simulink model "modello_carroponte_controllo"  (R2023b)
settings: Solver=FixedStepAuto  StartTime=0  StopTime=30  FixedStep=1e-3  RelTol=1e-3  EnableMultiTasking=on
values from neighbouring files (symbols this model uses):
  alpha_0 = 80 * pi/180    (= 1.3962634016)    [carroponte_controllo.m]
  alpha_dot_0 = 0    [carroponte_controllo.m]
  C = 5000 * Numerator/Denominator    [carroponte_controllo.m]
  cc = 5000    [carroponte_controllo.m]
  cm = 100    [carroponte_controllo.m]
  g = 9.81    [carroponte_controllo.m]
  L = 2.5    [carroponte_controllo.m]
  mc = 300    [carroponte_controllo.m]
  mm = 1000    [carroponte_controllo.m]
  xc_0 = 0    [carroponte_controllo.m]
  xc_dot_0 = 0    [carroponte_controllo.m]
libraries: slpidlib x1
settings Model: Creator=Gianmarco Rallo  LastModifiedBy=andrearosini
settings SolverCC: AlgebraicLoopSolver=TrustRegion
settings DataIOCC: LimitDataPoints=on  ReturnWorkspaceOutputs=off
settings OptimizationCC: BlockReduction=off  DefaultParameterBehavior=Inlined  BufferReuse=off  LifeSpan=inf
settings DebuggingCC: UnconnectedInputMsg=warning  UnconnectedOutputMsg=warning  UnconnectedLineMsg=warning  AllowSymbolicDim=off  SFUnexpectedBacktrackingDiag=warning  SFNoUnconditionalDefaultTransitionDiag=warning  SFExecutionAtInitializationDiag=none  ArithmeticOperatorsInVariantConditions=warning
settings ModelReferenceCC: EnableRefExpFcnMdlSchedulingChecks=on  PropagateSignalLabelsOutOfModel=off
settings SFSimCC: SimUseLocalCustomCode=off  CustomCodeUndefinedFunction=UseInterfaceOnly
settings RTWCC: RTWUseLocalCustomCode=off
settings CodeAppCC: StateflowObjectComments=on
settings GRTTargetCC: TargetLangStandard=C89/C90 (ANSI)
settings ConfigComp: CovMetricSettings=dw  CovSaveCumulativeToWorkspaceVar=on  CovSaveSingleToWorkspaceVar=on  CovExternalEMLEnable=off

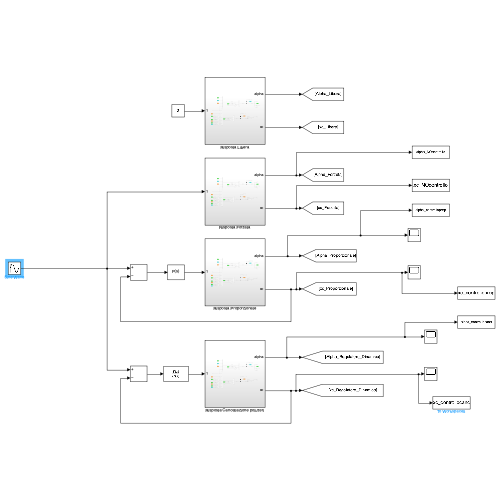
[thumbnail: Simulink's stored preview of the top-level diagram]
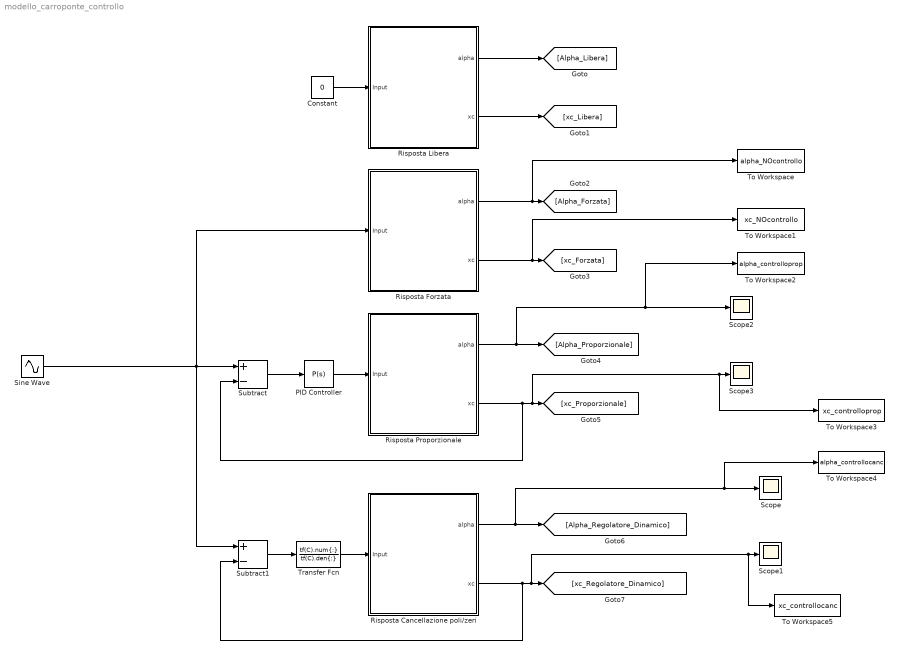
== system modello_carroponte_controllo ==
  Constant : Constant  Value=0
  PID Controller : slpidlib/PID Controller  Controller=P  Form=Parallel  TimeDomain=Continuous-time  UseExternalTs=off  SampleTime=-1  IntegratorMethod=Forward Euler  FilterMethod=Forward Euler  ControllerParametersSource=internal  P=5e3  I=1  UseKiTs=off  D=0  N=100  UseFilter=on  TunerSelectOption=Transfer Function Based (PID Tuner App)  InitialConditionSource=internal  InitialConditionForIntegrator=0  InitialConditionForFilter=0  DifferentiatorICPrevScaledInput=0  ExternalReset=none  TrackingMode=off  Kt=1  LimitOutput=off  SatLimitsSource=internal  UpperSaturationLimit=inf  LowerSaturationLimit=-inf  LinearizeAsGain=on  AntiWindupMode=none  Kb=1  LimitIntegrator=off  UpperIntegratorSaturationLimit=inf  LowerIntegratorSaturationLimit=-inf  POutMin=[]  POutMax=[]  IOutMin=[]  IOutMax=[]  DOutMin=[]  DOutMax=[]  NOutMin=[]  NOutMax=[]  SumOutMin=[]  SumOutMax=[]  SaturationOutMin=[]  SaturationOutMax=[]  PParamMin=[]  PParamMax=[]  IParamMin=[]  IParamMax=[]  DParamMin=[]  DParamMax=[]  NParamMin=[]  NParamMax=[]  KbParamMin=[]  KbParamMax=[]  KtParamMin=[]  KtParamMax=[]  KbOutMin=[]  KbOutMax=[]  KtOutMin=[]  KtOutMax=[]  IntegratorOutMin=[]  IntegratorOutMax=[]  FilterOutMin=[]  FilterOutMax=[]  SumI1OutMin=[]  SumI1OutMax=[]  SumI2OutMin=[]  SumI2OutMax=[]  SumI3OutMin=[]  SumI3OutMax=[]  SumI4OutMin=[]  SumI4OutMax=[]  SumDOutMin=[]  SumDOutMax=[]  DifferentiatorOutMin=[]  DifferentiatorOutMax=[]  FilterDiffOutCoefMin=[]  FilterDiffOutCoefMax=[]  ReciprocalOutMin=[]  ReciprocalOutMax=[]  SumDenOutMin=[]  SumDenOutMax=[]  SumNumOutMin=[]  SumNumOutMax=[]  DivideOutMin=[]  DivideOutMax=[]  UdiffTsProdOutMin=[]  UdiffTsProdOutMax=[]  NTsProdOutMin=[]  NTsProdOutMax=[]  UintegralTsProdOutMin=[]  UintegralTsProdOutMax=[]  UngainTsProdOutMin=[]  UngainTsProdOutMax=[]  ClampingZeroOutDataTypeStr=Inherit: Inherit via back propagation  ClampingZeroOutMin=[]  ClampingZeroOutMax=[]  FilterDenConstantOutDataTypeStr=Inherit: Inherit via back propagation  FilterDenConstantOutMin=[]  FilterDenConstantOutMax=[]  PCopyOutDataTypeStr=Inherit: Inherit via back propagation  PCopyOutMin=[]  PCopyOutMax=[]  NCopyOutDataTypeStr=Inherit: Inherit via back propagation  NCopyOutMin=[]  NCopyOutMax=[]  IntegratorContinuousStateAttributes=''  IntegratorStateMustResolveToSignalObject=off  IntegratorRTWStateStorageClass=Auto  FilterContinuousStateAttributes=''  FilterStateMustResolveToSignalObject=off  FilterRTWStateStorageClass=Auto  ParallelPVariant=InternalParameters  IdealPVariant=Disabled  IVariant=Disabled  DVariant=Disabled  IntegratorVariant=Disabled  SatVariant=Disabled  AWVariant=Disabled  PCopyVariant=Disabled  TRVariant=Disabled  FdbkBlocksVariant=Forward  IdealPFdbkVariant=Disabled  SatFdbkVariant=Disabled  DerivativeFilterVariant=Disabled  NVariant=Disabled  NCopyVariant=Disabled_SignalSpec  FilterICVariant=Disabled  IntegratorICVariant=Disabled  ExternalResetVariant=Disabled  TRSumVariant=Passthrough  SumFdbkVariant=Disabled  SumVariant=Passthrough_P  TsampFilterVariant=InternalTs  TsampNgainVariant=Passthrough  TsampIntegralVariant=Disabled_SignalSpec  ExternalSaturationOutDataTypeStr=Inherit: Same as second input
  Risposta Cancellazione poli/zeri : Subsystem
  Risposta Forzata : Subsystem
  Risposta Libera : Subsystem
  Risposta Proporzionale : Subsystem
  Scope{,1..3} (4 alike) : Scope
  Sine Wave : Sin  Amplitude=0  Frequency=2  SampleTime=0
  Subtract : Sum  Inputs=+-
  Subtract1 : Sum  Inputs=+-
  To Workspace : ToWorkspace  VariableName=alpha_NOcontrollo  SaveFormat=Timeseries  SampleTime=-1
  To Workspace1 : ToWorkspace  VariableName=xc_NOcontrollo  SaveFormat=Timeseries  SampleTime=-1
  To Workspace2 : ToWorkspace  VariableName=alpha_controlloprop  SaveFormat=Timeseries  SampleTime=-1
  To Workspace3 : ToWorkspace  VariableName=xc_controlloprop  SaveFormat=Timeseries  SampleTime=-1
  To Workspace4 : ToWorkspace  VariableName=alpha_controllocanc  SaveFormat=Timeseries  SampleTime=-1
  To Workspace5 : ToWorkspace  VariableName=xc_controllocanc  SaveFormat=Timeseries  SampleTime=-1
  Transfer Fcn : TransferFcn  Numerator=tf(C).num{:}  Denominator=tf(C).den{:}
  wires:
  Risposta Libera/1(alpha) -> [Alpha_Libera]
  Risposta Libera/2(xc) -> [xc_Libera]
  Constant/1 -> Risposta Libera/1(Input)
  Risposta Forzata/2(xc) -> To Workspace1/1, [xc_Forzata]
  Risposta Forzata/1(alpha) -> To Workspace/1, [Alpha_Forzata]
  Risposta Proporzionale/1(alpha) -> To Workspace2/1, Scope2/1, [Alpha_Proporzionale]
  Risposta Proporzionale/2(xc) -> Subtract/2, To Workspace3/1, Scope3/1, [xc_Proporzionale]
  PID Controller/1 -> Risposta Proporzionale/1(Input)
  Subtract/1 -> PID Controller/1
  Sine Wave/1 -> Risposta Forzata/1(Input), Subtract1/1, Subtract/1
  Subtract1/1 -> Transfer Fcn/1
  Transfer Fcn/1 -> Risposta Cancellazione poli/zeri/1(Input)
  Risposta Cancellazione poli/zeri/2(xc) -> To Workspace5/1, Scope1/1, [xc_Regolatore_Dinamico], Subtract1/2
  Risposta Cancellazione poli/zeri/1(alpha) -> To Workspace4/1, Scope/1, [Alpha_Regolatore_Dinamico]

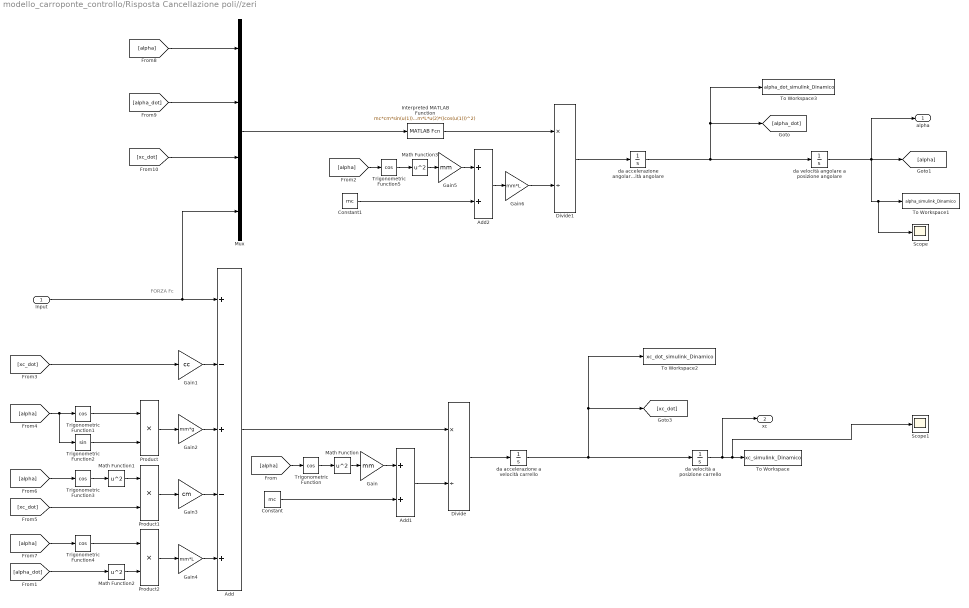
== system modello_carroponte_controllo/Risposta Cancellazione poli//zeri ==
  note: FORZA Fc
  Input : Inport
  Add : Sum  Inputs=+-+-+
  Add1 : Sum
  Add2 : Sum
  Constant : Constant  Value=mc
  Constant1 : Constant  Value=mc
  Divide : Product  Inputs=*/
  Divide1 : Product  Inputs=*/
  Gain : Gain  Gain=mm
  Gain1 : Gain  Gain=cc
  Gain2 : Gain  Gain=mm*g
  Gain3 : Gain  Gain=cm
  Gain4 : Gain  Gain=mm*L
  Gain5 : Gain  Gain=mm
  Gain6 : Gain  Gain=mm*L
  Interpreted MATLAB Function : MATLABFcn  MATLABFcn=mc*cm*sin(u(1))*u(3) - mm*cc*sin(u(1))*u(3) + (mm^2)*L*sin(u(1))*cos(u(1))*(u(2)^2) + mm*sin(u(1))*u(4) + (mm^2)*g*cos(u(1)) + mc*mm*g*cos(u(1)) - mc*cm*L*u(2) - mm*cm*L*u(2)*((cos(u(1)))^2)  OutputDimensions=1
  Math Function{,1..3} (4 alike) : Math  Operator=square  SignedPower=on
  Mux : Mux
  Product : Product
  Product1 : Product
  Product2 : Product
  Scope : Scope
  Scope1 : Scope
  To Workspace : ToWorkspace  VariableName=xc_simulink_Dinamico  SampleTime=-1
  To Workspace1 : ToWorkspace  VariableName=alpha_simulink_Dinamico  SampleTime=-1
  To Workspace2 : ToWorkspace  VariableName=xc_dot_simulink_Dinamico  SampleTime=-1
  To Workspace3 : ToWorkspace  VariableName=alpha_dot_simulink_Dinamico  SampleTime=-1
  Trigonometric Function{,1,3..5} (5 alike) : Trigonometry  Operator=cos
  Trigonometric Function2 : Trigonometry
  da accelerazione a velocità carrello : Integrator  InitialCondition=xc_dot_0
  da accelerazione angolare a velocità angolare : Integrator  InitialCondition=alpha_dot_0
  da velocità a posizione carrello : Integrator  InitialCondition=xc_0
  da velocità angolare a posizione angolare : Integrator  InitialCondition=alpha_0
  alpha : Outport
  xc : Outport  Port=2
  wires:
  Math Function2/1 -> Product2/2
  [alpha] -> Trigonometric Function4/1
  Gain4/1 -> Add/5
  [xc_dot] -> Mux/3
  Trigonometric Function3/1 -> Math Function1/1
  [alpha_dot] -> Math Function2/1
  Gain3/1 -> Add/4
  Product1/1 -> Gain3/1
  Gain6/1 -> Divide1/2
  Gain2/1 -> Add/3
  Divide/1 -> da accelerazione a velocità carrello/1
  [alpha_dot] -> Mux/2
  Input/1 -> Add/1, Mux/4
  [xc_dot] -> Gain1/1
  da velocità a posizione carrello/1 -> To Workspace/1, Scope1/1, xc/1
  Product2/1 -> Gain4/1
  Trigonometric Function/1 -> Math Function/1
  Product/1 -> Gain2/1
  Add2/1 -> Gain6/1
  Divide1/1 -> da accelerazione angolare a velocità angolare/1
  Interpreted MATLAB Function/1 -> Divide1/1
  Trigonometric Function4/1 -> Product2/1
  Gain5/1 -> Add2/1
  Trigonometric Function1/1 -> Product/1
  [alpha] -> Trigonometric Function5/1
  Gain1/1 -> Add/2
  Trigonometric Function5/1 -> Math Function3/1
  Add1/1 -> Divide/2
  Constant1/1 -> Add2/2
  Add/1 -> Divide/1
  Math Function3/1 -> Gain5/1
  Mux/1 -> Interpreted MATLAB Function/1
  Constant/1 -> Add1/2
  [alpha] -> Trigonometric Function1/1, Trigonometric Function2/1
  [xc_dot] -> Product1/2
  Math Function1/1 -> Product1/1
  Trigonometric Function2/1 -> Product/2
  da accelerazione angolare a velocità angolare/1 -> da velocità angolare a posizione angolare/1, [alpha_dot], To Workspace3/1
  [alpha] -> Trigonometric Function/1
  da accelerazione a velocità carrello/1 -> [xc_dot], To Workspace2/1, da velocità a posizione carrello/1
  [alpha] -> Mux/1
  [alpha] -> Trigonometric Function3/1
  Math Function/1 -> Gain/1
  Gain/1 -> Add1/1
  da velocità angolare a posizione angolare/1 -> [alpha], To Workspace1/1, Scope/1, alpha/1

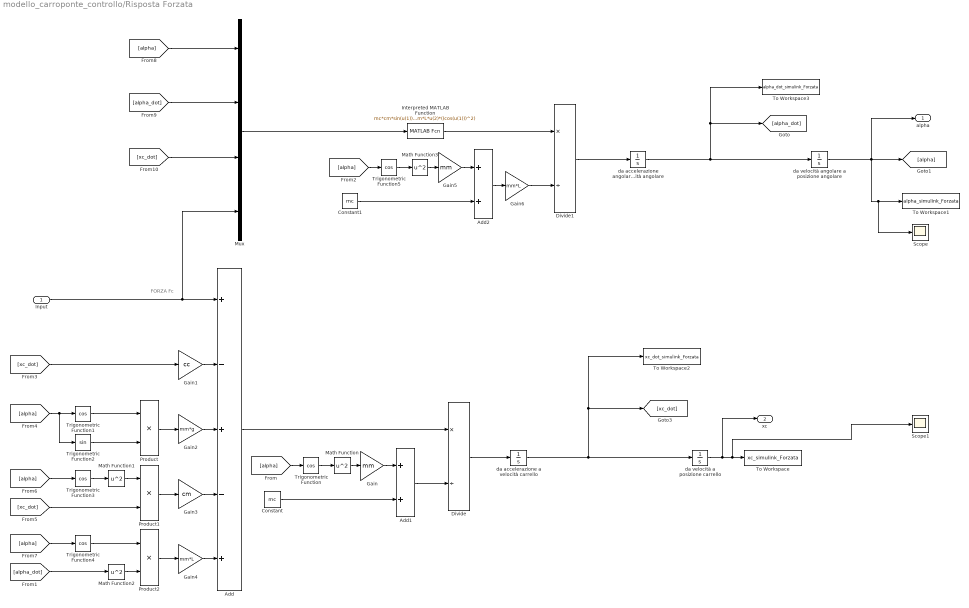
== system modello_carroponte_controllo/Risposta Forzata ==
  note: FORZA Fc
  Input : Inport
  Add : Sum  Inputs=+-+-+
  Add1 : Sum
  Add2 : Sum
  Constant : Constant  Value=mc
  Constant1 : Constant  Value=mc
  Divide : Product  Inputs=*/
  Divide1 : Product  Inputs=*/
  Gain : Gain  Gain=mm
  Gain1 : Gain  Gain=cc
  Gain2 : Gain  Gain=mm*g
  Gain3 : Gain  Gain=cm
  Gain4 : Gain  Gain=mm*L
  Gain5 : Gain  Gain=mm
  Gain6 : Gain  Gain=mm*L
  Interpreted MATLAB Function : MATLABFcn  MATLABFcn=mc*cm*sin(u(1))*u(3) - mm*cc*sin(u(1))*u(3) + (mm^2)*L*sin(u(1))*cos(u(1))*(u(2)^2) + mm*sin(u(1))*u(4) + (mm^2)*g*cos(u(1)) + mc*mm*g*cos(u(1)) - mc*cm*L*u(2) - mm*cm*L*u(2)*((cos(u(1)))^2)  OutputDimensions=1
  Math Function{,1..3} (4 alike) : Math  Operator=square  SignedPower=on
  Mux : Mux
  Product : Product
  Product1 : Product
  Product2 : Product
  Scope : Scope
  Scope1 : Scope
  To Workspace : ToWorkspace  VariableName=xc_simulink_Forzata  SampleTime=-1
  To Workspace1 : ToWorkspace  VariableName=alpha_simulink_Forzata  SampleTime=-1
  To Workspace2 : ToWorkspace  VariableName=xc_dot_simulink_Forzata  SampleTime=-1
  To Workspace3 : ToWorkspace  VariableName=alpha_dot_simulink_Forzata  SampleTime=-1
  Trigonometric Function{,1,3..5} (5 alike) : Trigonometry  Operator=cos
  Trigonometric Function2 : Trigonometry
  da accelerazione a velocità carrello : Integrator  InitialCondition=xc_dot_0
  da accelerazione angolare a velocità angolare : Integrator  InitialCondition=alpha_dot_0
  da velocità a posizione carrello : Integrator  InitialCondition=xc_0
  da velocità angolare a posizione angolare : Integrator  InitialCondition=alpha_0
  alpha : Outport
  xc : Outport  Port=2
  wires:
  Math Function2/1 -> Product2/2
  [alpha] -> Trigonometric Function4/1
  Gain4/1 -> Add/5
  [xc_dot] -> Mux/3
  Trigonometric Function3/1 -> Math Function1/1
  [alpha_dot] -> Math Function2/1
  Gain3/1 -> Add/4
  Product1/1 -> Gain3/1
  Gain6/1 -> Divide1/2
  Gain2/1 -> Add/3
  Divide/1 -> da accelerazione a velocità carrello/1
  [alpha_dot] -> Mux/2
  Input/1 -> Add/1, Mux/4
  [xc_dot] -> Gain1/1
  da velocità a posizione carrello/1 -> To Workspace/1, Scope1/1, xc/1
  Product2/1 -> Gain4/1
  Trigonometric Function/1 -> Math Function/1
  Product/1 -> Gain2/1
  Add2/1 -> Gain6/1
  Divide1/1 -> da accelerazione angolare a velocità angolare/1
  Interpreted MATLAB Function/1 -> Divide1/1
  Trigonometric Function4/1 -> Product2/1
  Gain5/1 -> Add2/1
  Trigonometric Function1/1 -> Product/1
  [alpha] -> Trigonometric Function5/1
  Gain1/1 -> Add/2
  Trigonometric Function5/1 -> Math Function3/1
  Add1/1 -> Divide/2
  Constant1/1 -> Add2/2
  Add/1 -> Divide/1
  Math Function3/1 -> Gain5/1
  Mux/1 -> Interpreted MATLAB Function/1
  Constant/1 -> Add1/2
  [alpha] -> Trigonometric Function1/1, Trigonometric Function2/1
  [xc_dot] -> Product1/2
  Math Function1/1 -> Product1/1
  Trigonometric Function2/1 -> Product/2
  da accelerazione angolare a velocità angolare/1 -> da velocità angolare a posizione angolare/1, [alpha_dot], To Workspace3/1
  [alpha] -> Trigonometric Function/1
  da accelerazione a velocità carrello/1 -> [xc_dot], To Workspace2/1, da velocità a posizione carrello/1
  [alpha] -> Mux/1
  [alpha] -> Trigonometric Function3/1
  Math Function/1 -> Gain/1
  Gain/1 -> Add1/1
  da velocità angolare a posizione angolare/1 -> [alpha], To Workspace1/1, Scope/1, alpha/1

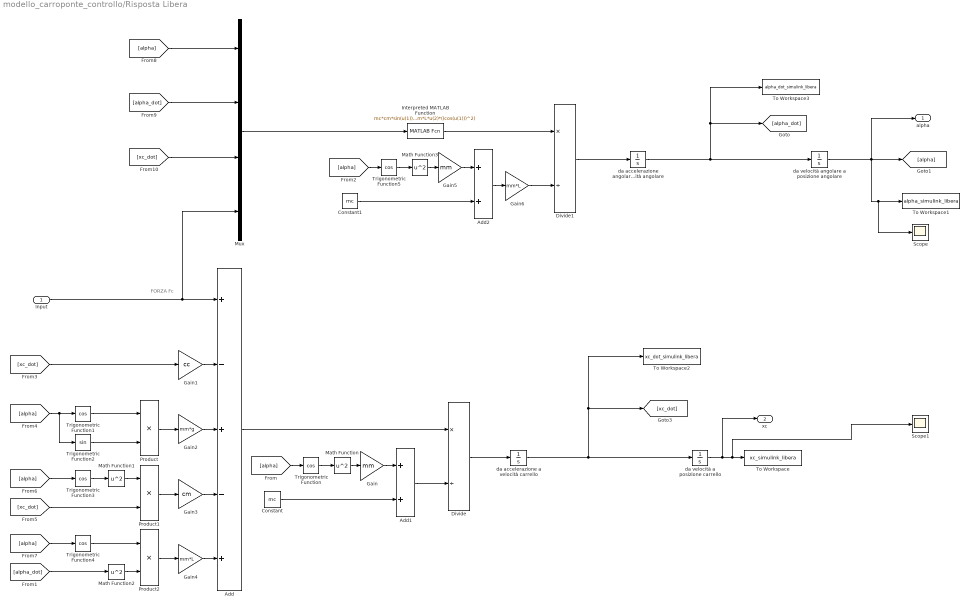
== system modello_carroponte_controllo/Risposta Libera ==
  note: FORZA Fc
  Input : Inport
  Add : Sum  Inputs=+-+-+
  Add1 : Sum
  Add2 : Sum
  Constant : Constant  Value=mc
  Constant1 : Constant  Value=mc
  Divide : Product  Inputs=*/
  Divide1 : Product  Inputs=*/
  Gain : Gain  Gain=mm
  Gain1 : Gain  Gain=cc
  Gain2 : Gain  Gain=mm*g
  Gain3 : Gain  Gain=cm
  Gain4 : Gain  Gain=mm*L
  Gain5 : Gain  Gain=mm
  Gain6 : Gain  Gain=mm*L
  Interpreted MATLAB Function : MATLABFcn  MATLABFcn=mc*cm*sin(u(1))*u(3) - mm*cc*sin(u(1))*u(3) + (mm^2)*L*sin(u(1))*cos(u(1))*(u(2)^2) + mm*sin(u(1))*u(4) + (mm^2)*g*cos(u(1)) + mc*mm*g*cos(u(1)) - mc*cm*L*u(2) - mm*cm*L*u(2)*((cos(u(1)))^2)  OutputDimensions=1
  Math Function{,1..3} (4 alike) : Math  Operator=square  SignedPower=on
  Mux : Mux
  Product : Product
  Product1 : Product
  Product2 : Product
  Scope : Scope
  Scope1 : Scope
  To Workspace : ToWorkspace  VariableName=xc_simulink_libera  SampleTime=-1
  To Workspace1 : ToWorkspace  VariableName=alpha_simulink_libera  SampleTime=-1
  To Workspace2 : ToWorkspace  VariableName=xc_dot_simulink_libera  SampleTime=-1
  To Workspace3 : ToWorkspace  VariableName=alpha_dot_simulink_libera  SampleTime=-1
  Trigonometric Function{,1,3..5} (5 alike) : Trigonometry  Operator=cos
  Trigonometric Function2 : Trigonometry
  da accelerazione a velocità carrello : Integrator  InitialCondition=xc_dot_0
  da accelerazione angolare a velocità angolare : Integrator  InitialCondition=alpha_dot_0
  da velocità a posizione carrello : Integrator  InitialCondition=xc_0
  da velocità angolare a posizione angolare : Integrator  InitialCondition=alpha_0
  alpha : Outport
  xc : Outport  Port=2
  wires:
  da velocità angolare a posizione angolare/1 -> alpha/1, Scope/1, To Workspace1/1, [alpha]
  Gain/1 -> Add1/1
  Math Function/1 -> Gain/1
  [alpha] -> Trigonometric Function3/1
  [alpha] -> Mux/1
  da accelerazione a velocità carrello/1 -> da velocità a posizione carrello/1, To Workspace2/1, [xc_dot]
  [alpha] -> Trigonometric Function/1
  da accelerazione angolare a velocità angolare/1 -> To Workspace3/1, [alpha_dot], da velocità angolare a posizione angolare/1
  Trigonometric Function2/1 -> Product/2
  Math Function1/1 -> Product1/1
  [xc_dot] -> Product1/2
  [alpha] -> Trigonometric Function2/1, Trigonometric Function1/1
  Constant/1 -> Add1/2
  Mux/1 -> Interpreted MATLAB Function/1
  Math Function3/1 -> Gain5/1
  Add/1 -> Divide/1
  Constant1/1 -> Add2/2
  Add1/1 -> Divide/2
  Trigonometric Function5/1 -> Math Function3/1
  Gain1/1 -> Add/2
  [alpha] -> Trigonometric Function5/1
  Trigonometric Function1/1 -> Product/1
  Gain5/1 -> Add2/1
  Trigonometric Function4/1 -> Product2/1
  Interpreted MATLAB Function/1 -> Divide1/1
  Divide1/1 -> da accelerazione angolare a velocità angolare/1
  Add2/1 -> Gain6/1
  Product/1 -> Gain2/1
  Trigonometric Function/1 -> Math Function/1
  Product2/1 -> Gain4/1
  da velocità a posizione carrello/1 -> xc/1, Scope1/1, To Workspace/1
  [xc_dot] -> Gain1/1
  Input/1 -> Mux/4, Add/1
  [alpha_dot] -> Mux/2
  Divide/1 -> da accelerazione a velocità carrello/1
  Gain2/1 -> Add/3
  Gain6/1 -> Divide1/2
  Product1/1 -> Gain3/1
  Gain3/1 -> Add/4
  [alpha_dot] -> Math Function2/1
  Trigonometric Function3/1 -> Math Function1/1
  [xc_dot] -> Mux/3
  Gain4/1 -> Add/5
  [alpha] -> Trigonometric Function4/1
  Math Function2/1 -> Product2/2

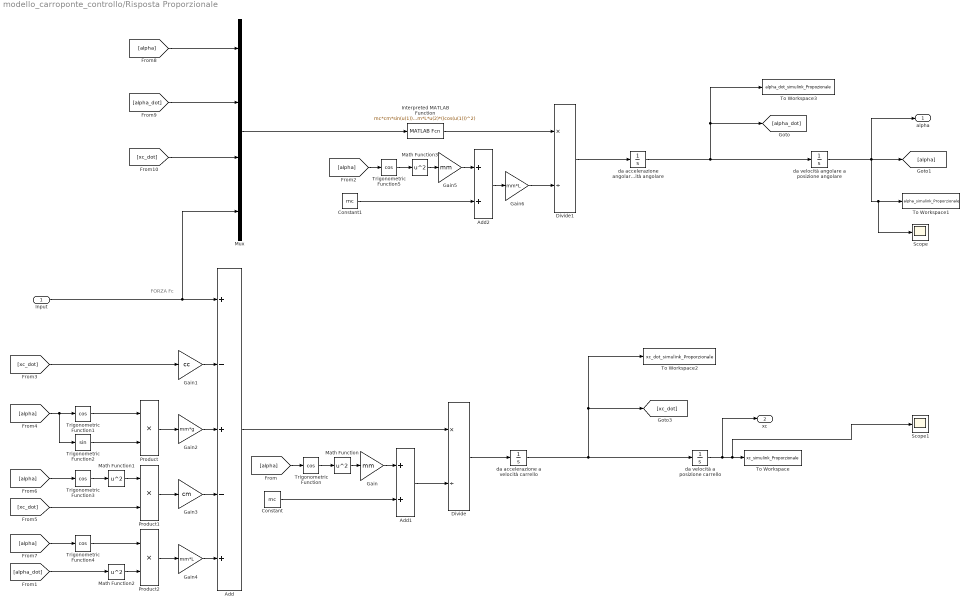
== system modello_carroponte_controllo/Risposta Proporzionale ==
  note: FORZA Fc
  Input : Inport
  Add : Sum  Inputs=+-+-+
  Add1 : Sum
  Add2 : Sum
  Constant : Constant  Value=mc
  Constant1 : Constant  Value=mc
  Divide : Product  Inputs=*/
  Divide1 : Product  Inputs=*/
  Gain : Gain  Gain=mm
  Gain1 : Gain  Gain=cc
  Gain2 : Gain  Gain=mm*g
  Gain3 : Gain  Gain=cm
  Gain4 : Gain  Gain=mm*L
  Gain5 : Gain  Gain=mm
  Gain6 : Gain  Gain=mm*L
  Interpreted MATLAB Function : MATLABFcn  MATLABFcn=mc*cm*sin(u(1))*u(3) - mm*cc*sin(u(1))*u(3) + (mm^2)*L*sin(u(1))*cos(u(1))*(u(2)^2) + mm*sin(u(1))*u(4) + (mm^2)*g*cos(u(1)) + mc*mm*g*cos(u(1)) - mc*cm*L*u(2) - mm*cm*L*u(2)*((cos(u(1)))^2)  OutputDimensions=1
  Math Function{,1..3} (4 alike) : Math  Operator=square  SignedPower=on
  Mux : Mux
  Product : Product
  Product1 : Product
  Product2 : Product
  Scope : Scope
  Scope1 : Scope
  To Workspace : ToWorkspace  VariableName=xc_simulink_Proporzionale  SampleTime=-1
  To Workspace1 : ToWorkspace  VariableName=alpha_simulink_Proporzionale  SampleTime=-1
  To Workspace2 : ToWorkspace  VariableName=xc_dot_simulink_Proporzionale  SampleTime=-1
  To Workspace3 : ToWorkspace  VariableName=alpha_dot_simulink_Propozionale  SampleTime=-1
  Trigonometric Function{,1,3..5} (5 alike) : Trigonometry  Operator=cos
  Trigonometric Function2 : Trigonometry
  da accelerazione a velocità carrello : Integrator  InitialCondition=xc_dot_0
  da accelerazione angolare a velocità angolare : Integrator  InitialCondition=alpha_dot_0
  da velocità a posizione carrello : Integrator  InitialCondition=xc_0
  da velocità angolare a posizione angolare : Integrator  InitialCondition=alpha_0
  alpha : Outport
  xc : Outport  Port=2
  wires:
  da velocità angolare a posizione angolare/1 -> alpha/1, Scope/1, To Workspace1/1, [alpha]
  Gain/1 -> Add1/1
  Math Function/1 -> Gain/1
  [alpha] -> Trigonometric Function3/1
  [alpha] -> Mux/1
  da accelerazione a velocità carrello/1 -> da velocità a posizione carrello/1, To Workspace2/1, [xc_dot]
  [alpha] -> Trigonometric Function/1
  da accelerazione angolare a velocità angolare/1 -> To Workspace3/1, [alpha_dot], da velocità angolare a posizione angolare/1
  Trigonometric Function2/1 -> Product/2
  Math Function1/1 -> Product1/1
  [xc_dot] -> Product1/2
  [alpha] -> Trigonometric Function2/1, Trigonometric Function1/1
  Constant/1 -> Add1/2
  Mux/1 -> Interpreted MATLAB Function/1
  Math Function3/1 -> Gain5/1
  Add/1 -> Divide/1
  Constant1/1 -> Add2/2
  Add1/1 -> Divide/2
  Trigonometric Function5/1 -> Math Function3/1
  Gain1/1 -> Add/2
  [alpha] -> Trigonometric Function5/1
  Trigonometric Function1/1 -> Product/1
  Gain5/1 -> Add2/1
  Trigonometric Function4/1 -> Product2/1
  Interpreted MATLAB Function/1 -> Divide1/1
  Divide1/1 -> da accelerazione angolare a velocità angolare/1
  Add2/1 -> Gain6/1
  Product/1 -> Gain2/1
  Trigonometric Function/1 -> Math Function/1
  Product2/1 -> Gain4/1
  da velocità a posizione carrello/1 -> xc/1, Scope1/1, To Workspace/1
  [xc_dot] -> Gain1/1
  Input/1 -> Mux/4, Add/1
  [alpha_dot] -> Mux/2
  Divide/1 -> da accelerazione a velocità carrello/1
  Gain2/1 -> Add/3
  Gain6/1 -> Divide1/2
  Product1/1 -> Gain3/1
  Gain3/1 -> Add/4
  [alpha_dot] -> Math Function2/1
  Trigonometric Function3/1 -> Math Function1/1
  [xc_dot] -> Mux/3
  Gain4/1 -> Add/5
  [alpha] -> Trigonometric Function4/1
  Math Function2/1 -> Product2/2
